simulink model "Modelos"  (Simulink 8.0)
settings: Solver=VariableStepDiscrete  StartTime=0.0  StopTime=10.0  MaxStep=0.06  RelTol=1e-3
values from neighbouring files (symbols this model uses):
  radio = 0.1    [matlab.mat]
undefined symbols (not defined in the file or in its folder): DiscIntNeverNeededParam
libraries: simulink x4
settings Model: Creator=borJaRal  LastModifiedBy=borJaRal

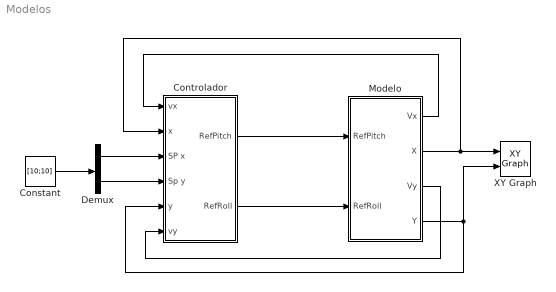
== system Modelos ==
  " Modelo" : Subsystem
  Constant : Constant  Value=[10;10]  SampleTime=0.06
  Controlador : Subsystem
  Demux : Demux  Outputs=2
  XY Graph : simulink/Sinks/XY Graph  xmin=-15  xmax=20  ymin=-10  ymax=15  st=0.06
  wires:
  " Modelo"/2(X) -> XY Graph/1, Controlador/2(x)
  " Modelo"/4(Y) -> Controlador/5(y), XY Graph/2
  Controlador/1(RefPitch) -> " Modelo"/1(RefPitch)
  Controlador/2(RefRoll) -> " Modelo"/2(RefRoll)
  " Modelo"/1(Vx) -> Controlador/1(vx)
  " Modelo"/3(Vy) -> Controlador/6(vy)
  Demux/1 -> Controlador/3(SP x)
  Demux/2 -> Controlador/4(Sp y)
  Constant/1 -> Demux/1

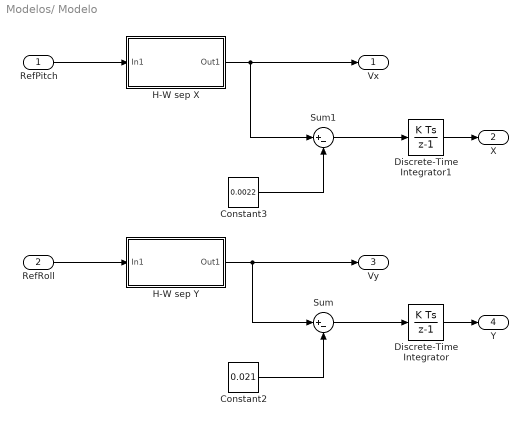
== system Modelos/ Modelo ==
  RefPitch : Inport  PortDimensions=1  SampleTime=0.06
  RefRoll : Inport  Port=2  PortDimensions=1  SampleTime=0.06
  Constant2 : Constant  Value=0.021
  Constant3 : Constant  Value=0.0022
  Discrete-Time Integrator : DiscreteIntegrator  gainval=0.95  InitialCondition=-1  SampleTime=0.06  ICPrevOutput=DiscIntNeverNeededParam  ICPrevScaledInput=DiscIntNeverNeededParam
  Discrete-Time Integrator1 : DiscreteIntegrator  gainval=1  SampleTime=0.06  ICPrevOutput=DiscIntNeverNeededParam  ICPrevScaledInput=DiscIntNeverNeededParam
  H-W sep X : Subsystem
  H-W sep Y : Subsystem
  Sum : Sum  Inputs=|+-
  Sum1 : Sum  Inputs=|+-
  Vx : Outport
  X : Outport  Port=2
  Vy : Outport  Port=3
  Y : Outport  Port=4
  wires:
  H-W sep X/1(Out1) -> Sum1/1, Vx/1
  RefRoll/1 -> H-W sep Y/1(In1)
  RefPitch/1 -> H-W sep X/1(In1)
  Discrete-Time Integrator/1 -> Y/1
  Discrete-Time Integrator1/1 -> X/1
  H-W sep Y/1(Out1) -> Sum/1, Vy/1
  Sum/1 -> Discrete-Time Integrator/1
  Constant2/1 -> Sum/2
  Sum1/1 -> Discrete-Time Integrator1/1
  Constant3/1 -> Sum1/2

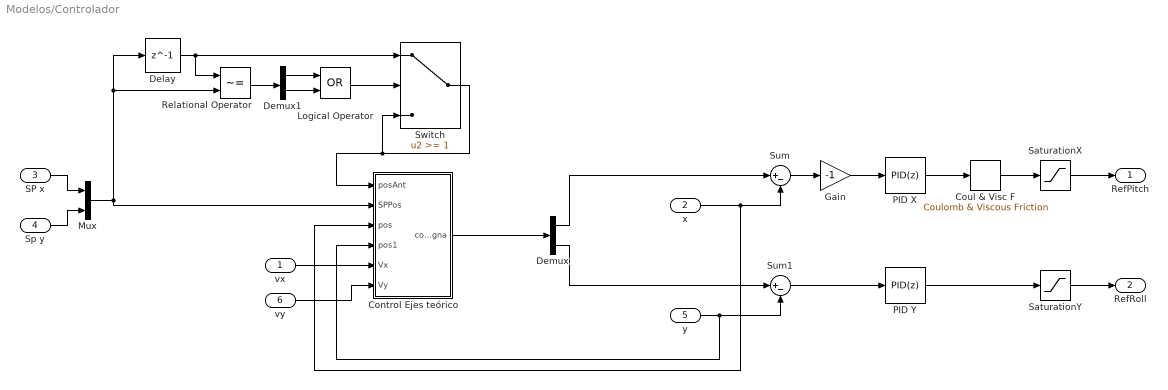
== system Modelos/Controlador ==
  vx : Inport
  x : Inport  Port=2
  SP x : Inport  Port=3
  Sp y : Inport  Port=4
  y : Inport  Port=5
  vy : Inport  Port=6
  Control Ejes teórico : Subsystem
  Coul & Visc F : simulink/Discontinuities/Coulomb & Viscous Friction  offset=0.07  gain=1
  Delay : Delay  DelayLength=1  InitialCondition=0  SampleTime=0.06
  Demux : Demux  Outputs=2
  Demux1 : Demux  Outputs=2
  Gain : Gain  Gain=-1  SampleTime=0.06
  Logical Operator : Logic  Operator=OR  AllPortsSameDT=off  OutDataTypeStr=boolean  SampleTime=0.06
  Mux : Mux  Inputs=2
  PID X : simulink/Continuous/PID Controller  Controller=PID  TimeDomain=Discrete-time  SampleTime=0.06  IntegratorMethod=Forward Euler  FilterMethod=Forward Euler  Form=Parallel  P=0.1  I=0  D=0.05  N=12  InitialConditionSource=internal  InitialConditionForIntegrator=0  InitialConditionForFilter=0  ExternalReset=none  LimitOutput=off  UpperSaturationLimit=inf  LowerSaturationLimit=-inf  LinearizeAsGain=off  AntiWindupMode=none  Kb=1  TrackingMode=off  Kt=1  PParamMin=[]  PParamMax=[]  IParamMin=[]  IParamMax=[]  DParamMin=[]  DParamMax=[]  NParamMin=[]  NParamMax=[]  KbParamMin=[]  KbParamMax=[]  KtParamMin=[]  KtParamMax=[]  POutMin=[]  POutMax=[]  IOutMin=[]  IOutMax=[]  DOutMin=[]  DOutMax=[]  NOutMin=[]  NOutMax=[]  KbOutMin=[]  KbOutMax=[]  KtOutMin=[]  KtOutMax=[]  IntegratorOutMin=[]  IntegratorOutMax=[]  FilterOutMin=[]  FilterOutMax=[]  SumOutMin=[]  SumOutMax=[]  SumI1OutMin=[]  SumI1OutMax=[]  SumI2OutMin=[]  SumI2OutMax=[]  SumI3OutMin=[]  SumI3OutMax=[]  SumDOutMin=[]  SumDOutMax=[]  SaturationOutMin=[]  SaturationOutMax=[]  IntegratorContinuousStateAttributes=''  IntegratorStateMustResolveToSignalObject=off  IntegratorRTWStateStorageClass=Auto  FilterContinuousStateAttributes=''  FilterStateMustResolveToSignalObject=off  FilterRTWStateStorageClass=Auto
  PID Y : simulink/Continuous/PID Controller  Controller=PID  TimeDomain=Discrete-time  SampleTime=0.06  IntegratorMethod=Forward Euler  FilterMethod=Forward Euler  Form=Parallel  P=1.5  I=0  D=3  N=20  InitialConditionSource=internal  InitialConditionForIntegrator=0  InitialConditionForFilter=0  ExternalReset=none  LimitOutput=off  UpperSaturationLimit=inf  LowerSaturationLimit=-inf  LinearizeAsGain=off  AntiWindupMode=none  Kb=1  TrackingMode=off  Kt=1  PParamMin=[]  PParamMax=[]  IParamMin=[]  IParamMax=[]  DParamMin=[]  DParamMax=[]  NParamMin=[]  NParamMax=[]  KbParamMin=[]  KbParamMax=[]  KtParamMin=[]  KtParamMax=[]  POutMin=[]  POutMax=[]  IOutMin=[]  IOutMax=[]  DOutMin=[]  DOutMax=[]  NOutMin=[]  NOutMax=[]  KbOutMin=[]  KbOutMax=[]  KtOutMin=[]  KtOutMax=[]  IntegratorOutMin=[]  IntegratorOutMax=[]  FilterOutMin=[]  FilterOutMax=[]  SumOutMin=[]  SumOutMax=[]  SumI1OutMin=[]  SumI1OutMax=[]  SumI2OutMin=[]  SumI2OutMax=[]  SumI3OutMin=[]  SumI3OutMax=[]  SumDOutMin=[]  SumDOutMax=[]  SaturationOutMin=[]  SaturationOutMax=[]  IntegratorContinuousStateAttributes=''  IntegratorStateMustResolveToSignalObject=off  IntegratorRTWStateStorageClass=Auto  FilterContinuousStateAttributes=''  FilterStateMustResolveToSignalObject=off  FilterRTWStateStorageClass=Auto
  Relational Operator : RelationalOperator  Operator=~=  OutDataTypeStr=boolean  SampleTime=0.06
  SaturationX : Saturate  UpperLimit=0.6  LowerLimit=-0.6  SampleTime=0.06
  SaturationY : Saturate  UpperLimit=0.6  LowerLimit=-0.65  SampleTime=0.06
  Sum : Sum  Inputs=|+-
  Sum1 : Sum  Inputs=|+-
  Switch : Switch  Threshold=1  SampleTime=0.06
  RefPitch : Outport
  RefRoll : Outport  Port=2
  wires:
  SaturationX/1 -> RefPitch/1
  x/1 -> Control Ejes teórico/3(pos), Sum/2
  Sum/1 -> Gain/1
  Gain/1 -> PID X/1
  SaturationY/1 -> RefRoll/1
  PID Y/1 -> SaturationY/1
  PID X/1 -> Coul & Visc F/1
  SP x/1 -> Mux/1
  Sp y/1 -> Mux/2
  Mux/1 -> Control Ejes teórico/2(SPPos), Delay/1, Relational Operator/2
  Control Ejes teórico/1(consigna) -> Demux/1
  y/1 -> Control Ejes teórico/4(pos1), Sum1/2
  Sum1/1 -> PID Y/1
  Demux/2 -> Sum1/1
  Demux/1 -> Sum/1
  Relational Operator/1 -> Demux1/1
  Delay/1 -> Relational Operator/1, Switch/1
  Switch/1 -> Control Ejes teórico/1(posAnt), Switch/3
  Demux1/1 -> Logical Operator/1
  Demux1/2 -> Logical Operator/2
  Logical Operator/1 -> Switch/2
  vx/1 -> Control Ejes teórico/5(Vx)
  vy/1 -> Control Ejes teórico/6(Vy)
  Coul & Visc F/1 -> SaturationX/1

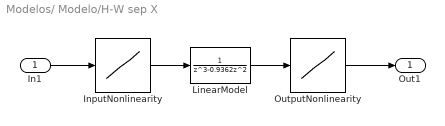
== system Modelos/ Modelo/H-W sep X ==
  In1 : Inport
  InputNonlinearity : Lookup_n-D  NumberOfTableDimensions=1  BreakpointsForDimension1=[-0.7794306773114486,-0.6665517461335803,-0.38259787912288773,-0.25092725123883536,0.09473639847108406,0.17029673563619527,0.17726636436631915,0.37957998009039323,0.38295482334780956,0.6895983704409222,0.7117318741228923,0.7447670914223733]  Table=[-0.5252577071737793,-0.5740314668184492,-0.5276067440181784,-0.4525234907735544,0.08939370174418115,0.1805352107680322,0.1868036147839089,0.3543585215551489,0.3611326480203565,0.37788310108320206,0.3526197208305561,0.3422075436511802]  RndMeth=Simplest  InputSameDT=on
  LinearModel : DiscreteTransferFcn  Denominator=[1 -0.9362 0 0]  SampleTime=0.06
  OutputNonlinearity : Lookup_n-D  NumberOfTableDimensions=1  BreakpointsForDimension1=[-13.100440261829927,-10.750187015480893,-9.470137574293718,-9.36690448652481,-6.389442383224805,-1.6138287974253407,-0.297953925902821,1.971981554283074,2.7910296318480756,5.162248586236924,10.40110370041321,12.751035076726279]  Table=[3.2664521299029508,3.5252407787384157,3.7330540769149074,3.7540914265089205,2.1259511153246806,-0.05999829191880518,0.057697690602710905,-1.1460016436590341,-1.5145126126505724,-3.1269313395607856,-4.168177689419741,-4.391972300120799]  RndMeth=Simplest  InputSameDT=on
  Out1 : Outport
  wires:
  In1/1 -> InputNonlinearity/1
  InputNonlinearity/1 -> LinearModel/1
  LinearModel/1 -> OutputNonlinearity/1
  OutputNonlinearity/1 -> Out1/1

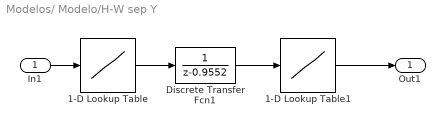
== system Modelos/ Modelo/H-W sep Y ==
  In1 : Inport
  1-D Lookup Table : Lookup_n-D  NumberOfTableDimensions=1  BreakpointsForDimension1=[-1.1225240009047588,-0.6108756671535277,-0.3128790658307752,-0.2913817412551785,0.00938351236428661,0.0677515420237256,0.16514140233265545,0.30042635723557465,0.3198218836765622,0.6045751627566303]  Table=[-0.5474321358905286,-0.6404833604115172,-0.42292715552017335,-0.5324214704084676,-0.07618732053051584,0.012562344805443028,0.16039796318878402,0.3172882429080992,0.23894258382025083,0.4664650461409855]  RndMeth=Simplest  InputSameDT=on
  1-D Lookup Table1 : Lookup_n-D  NumberOfTableDimensions=1  BreakpointsForDimension1=[-15.832778908250022,-13.7342083264422,-10.320129925856286,-7.501158359462719,-2.9390386213145105,-0.8462396811445138,3.4795365065330883,6.504839362526322,9.44668430471862,15.634316306375393]  Table=[-2.368387652340793,-2.140120269158168,-1.5133016751064454,-1.0738581735644925,0.03563887557433881,-0.012667991728073244,1.0709692692542954,1.5353474643531277,2.0716251012590496,2.127622896339377]  RndMeth=Simplest  InputSameDT=on
  Discrete Transfer Fcn1 : DiscreteTransferFcn  Denominator=[1 -0.9552]  SampleTime=0.06
  Out1 : Outport
  wires:
  In1/1 -> 1-D Lookup Table/1
  1-D Lookup Table1/1 -> Out1/1
  1-D Lookup Table/1 -> Discrete Transfer Fcn1/1
  Discrete Transfer Fcn1/1 -> 1-D Lookup Table1/1

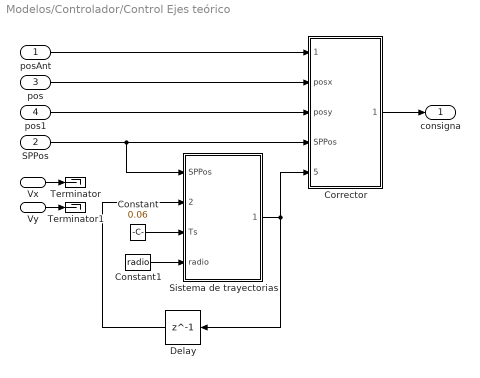
== system Modelos/Controlador/Control Ejes teórico ==
  posAnt : Inport
  SPPos : Inport  Port=2
  pos : Inport  Port=3
  pos1 : Inport  Port=4
  Vx : Inport  Port=5
  Vy : Inport  Port=6
  Constant : Constant  Value=0.06  SampleTime=0.06
  Constant1 : Constant  Value=radio  SampleTime=0.06
  Corrector : MATLAB Function  TreatAsAtomicUnit=on
  Delay : Delay  DelayLength=1  InitialCondition=0  SampleTime=0.06
  Sistema de trayectorias : MATLAB Function  TreatAsAtomicUnit=on  SystemSampleTime=0.06
  Terminator : Terminator
  Terminator1 : Terminator
  consigna : Outport
  wires:
  SPPos/1 -> Corrector/4(SPPos), Sistema de trayectorias/1(SPPos)
  Constant/1 -> Sistema de trayectorias/3(Ts)
  Constant1/1 -> Sistema de trayectorias/4(radio)
  posAnt/1 -> Corrector/1(posAnt)
  pos/1 -> Corrector/2(posx)
  Delay/1 -> Sistema de trayectorias/2(LastRef)
  Sistema de trayectorias/1(CurrRef) -> Delay/1, Corrector/5(CurrRef)
  Corrector/1(consigna) -> consigna/1
  pos1/1 -> Corrector/3(posy)
  Vx/1 -> Terminator/1
  Vy/1 -> Terminator1/1

== matlab function Controlador/Control Ejes teórico/Corrector ==
  data: posAnt input double; posx input double; posy input double; SPPos input double; CurrRef input double; consigna output double
function consigna = CalcRef(posAnt,posx,posy,SPPos,CurrRef)

A=posAnt;
B=SPPos;
C=[posx;posy]; %construimos vector posicion

% creamos vector director de la recta AB (recta r)
Vr = B-A;

% iniciamos vector Vs
Vs = Vr;

% creamos vector perpendicular a Vr
Vs(1,1) = -Vr(2,1);
Vs(2,1) = Vr(1,1);

% creamos matriz de vectores directores
MatrA = [Vr,-Vs];

% creamos matriz de valores independientes
MatrB = C-A;

% calculamos los valores de las K's de cada recta
K = inv(MatrA)*MatrB;

% sacamos el punto D intereseccion de las rectas
D = A + K(1,1)*Vr;

vE = D-C;

%% Calculo cuando CurrRef no está sobre la trayectoria
% Se añade esta segunda parte para corregir desviaciones de la trayectoria 
% ideal teórica de la forma apropiada y evitar discrepancias según el método 
% de gestión de consigna empleado. Funciona correctamente.

% creamos matriz de valores independientes
MatrC = CurrRef-A;

% calculamos los valores de las K's de cada recta
K1 = inv(MatrA)*MatrC;

% sacamos el punto E, vertical desde CurrRef, intereseccion de las rectas
% con trayectoria
E = A + K1(1,1)*Vr;
% Permite seleccionar el instante al que afecta la
% magnitud de la corrección (posible introducción a la corrección variable
% selectiva)
   if norm(vE)>0.5
           consigna = E + vE*10;
    else
        consigna = E + vE*3;
    end

== matlab function Controlador/Control Ejes teórico/Sistema de trayectorias ==
  data: CurrRef output double size=2; SPPos input double; LastRef input double; Ts input double; radio input double
function CurrRef = CalcRef(SPPos,LastRef,Ts,radio)
% Este bloque es un control de velocidad y aceleración a título teórico para
% definir las consignas a seguir según unas velocidades y aceleraciones
% máximas teóricas constantes obtenidas experimentalmente en los modelos.
% No corrige las imprecisiones en la trayectoria y el desincronismo de los ejes
% en el arranque. Problemas en la llegada de sobrepasamiento.

%% Valores límite calculados experimentalmente
maxVx = 2;
maxVy = 1;

%% Método de control simple

DistXY = SPPos-LastRef;

if (norm(DistXY)<(0.5*radio)) % (0.5*radio)
    CurrRef = SPPos;
else
    minTx = abs (DistXY(1))/maxVx;
    minTy = abs (DistXY(2))/maxVy;
    
    minT = max (minTx,minTy);
    
    if minT<Ts
        CurrRef = SPPos;
    else
        CurrRef = LastRef + (Ts/minT)*DistXY;
    end
end
